simulink model "example24"  (R2023b)
settings: Solver=ode45  StartTime=0.0  StopTime=200  MaxStep=0.01  RelTol=1e-6
settings Model: Creator=tom  LastModifiedBy=tom
settings SolverCC: ShapePreserveControl=EnableAll
settings ModelReferenceCC: EnableRefExpFcnMdlSchedulingChecks=on

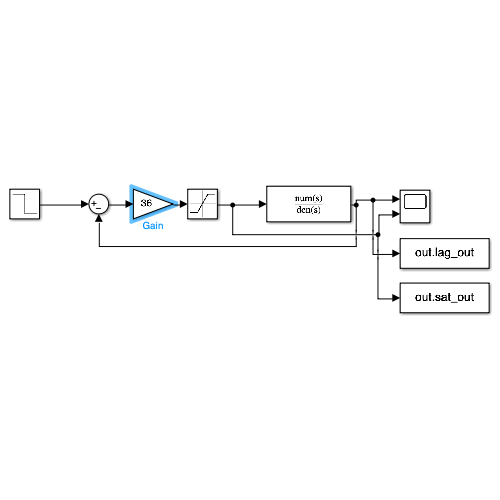
[thumbnail: Simulink's stored preview of the top-level diagram]
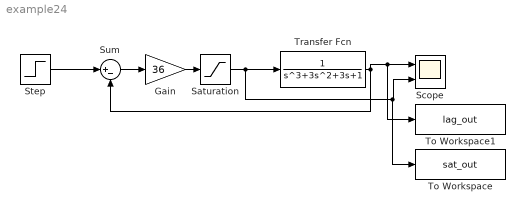
== system example24 ==
  Gain : Gain  Gain=36
  Saturation : Saturate  UpperLimit=1  LowerLimit=-1
  Scope : Scope  NumInputPorts=2
  Step : Step  Time=0.1  Before=1  After=0  SampleTime=0
  Sum : Sum  Inputs=|+-
  To Workspace : ToWorkspace  VariableName=sat_out  SampleTime=-1
  To Workspace1 : ToWorkspace  VariableName=lag_out  SampleTime=-1
  Transfer Fcn : TransferFcn  Denominator=[1 3 3 1]
  wires:
  Sum/1 -> Gain/1
  Transfer Fcn/1 -> To Workspace1/1, Scope/1, Sum/2
  Gain/1 -> Saturation/1
  Step/1 -> Sum/1
  Saturation/1 -> To Workspace/1, Scope/2, Transfer Fcn/1
